simulink model "simulator"  (R2022a)
settings: Solver=FixedStepAuto  StartTime=0.0  StopTime=inf  FixedStep=0.001  RelTol=1e-3
values from neighbouring files (symbols this model uses):
  PWM = [2000;2000;2000;2000]    [startup.m]
undefined symbols (not defined in the file or in its folder): Init, Motor, Vehicle
libraries: matrix_library x2, sldrtlib x1, aerolibnav x1, aerolibanimutils x1, shared6dof x1, sharedtransform x1
settings Model: Creator=Thana  LastModifiedBy=Thana

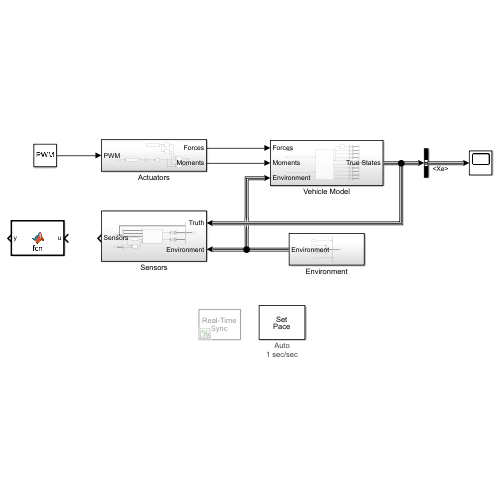
[thumbnail: Simulink's stored preview of the top-level diagram]
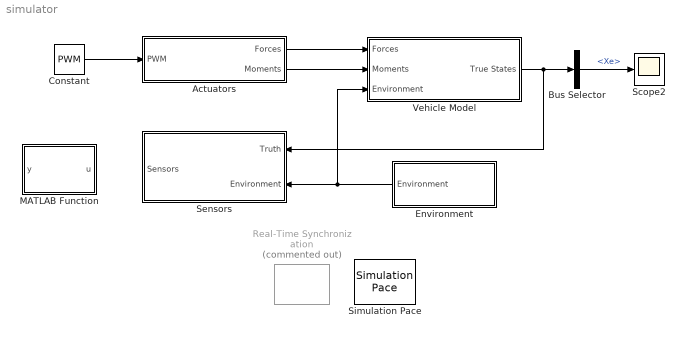
== system simulator ==
  Actuators : Subsystem
  Bus Selector : BusSelector  OutputSignals=Xe
  Constant : Constant  Value=PWM
  Environment : Subsystem
  MATLAB Function : MATLAB Function  TreatAsAtomicUnit=on
  Real-Time Synchronization : sldrtlib/Real-Time Synchronization  Commented=on  SampleTime=1  MaxMissedTicks=1000  ShowMissedTicks=off  YieldWhenWaiting=off
  Scope2 : Scope
  Sensors : Subsystem
  Simulation Pace : aerolibanimutils/Simulation Pace  SimulationPace=1  SleepMode=Auto  OutputPaceError=off  SampleTime=-1
  Vehicle Model : Subsystem
  wires:
  Vehicle Model/1(True States) -> Bus Selector/1, Sensors/1(Truth)
  Environment/1(Environment) -> Vehicle Model/3(Environment), Sensors/2(Environment)
  Actuators/2(Moments) -> Vehicle Model/2(Moments)
  Actuators/1(Forces) -> Vehicle Model/1(Forces)
  Constant/1 -> Actuators/1(PWM)
  Bus Selector/1 -> Scope2/1  "<Xe>"

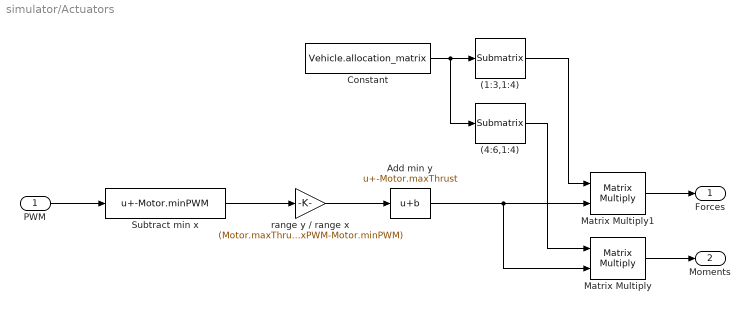
== system simulator/Actuators ==
  PWM : Inport
  (1:3,1:4) : matrix_library/Submatrix  RowSpan=Range of rows  RowStartMode=Index  RowStartIndex=1  RowEndMode=Index  RowEndIndex=3  ColSpan=Range of columns  ColStartMode=Index  ColStartIndex=1  ColEndMode=Index  ColEndIndex=4
      settings: SourceProductBaseCode=SL
  (4:6,1:4) : matrix_library/Submatrix  RowSpan=Range of rows  RowStartMode=Index  RowStartIndex=4  RowEndMode=Index  RowEndIndex=6  ColSpan=Range of columns  ColStartMode=Index  ColStartIndex=1  ColEndMode=Index  ColEndIndex=4
      settings: SourceProductBaseCode=SL
  Add min y : Bias  Bias=-Motor.maxThrust  SaturateOnIntegerOverflow=off
  Constant : Constant  Value=Vehicle.allocation_matrix
  Matrix Multiply : Product  Multiplication=Matrix(*)
  Matrix Multiply1 : Product  Multiplication=Matrix(*)
  Subtract min x : Bias  Bias=-Motor.minPWM  SaturateOnIntegerOverflow=off
  range y / range x : Gain  Gain=(Motor.maxThrust-(-Motor.maxThrust))./(Motor.maxPWM-Motor.minPWM)
  Forces : Outport
  Moments : Outport  Port=2
  wires:
  Add min y/1 -> Matrix Multiply1/2, Matrix Multiply/2
  Subtract min x/1 -> range y / range x/1
  PWM/1 -> Subtract min x/1
  range y / range x/1 -> Add min y/1
  Constant/1 -> (4:6,1:4)/1, (1:3,1:4)/1
  (4:6,1:4)/1 -> Matrix Multiply/1
  (1:3,1:4)/1 -> Matrix Multiply1/1
  Matrix Multiply1/1 -> Forces/1
  Matrix Multiply/1 -> Moments/1

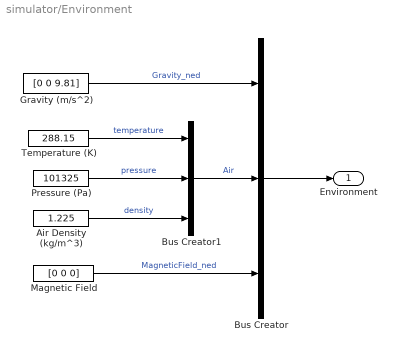
== system simulator/Environment ==
  Air Density (kg/m^3) : Constant  Value=1.225
  Bus Creator : BusCreator  Inputs=3
  Bus Creator1 : BusCreator  Inputs=3
  Gravity (m/s^2) : Constant  Value=[0 0 9.81]
  Magnetic Field : Constant  Value=[0 0 0]
  Pressure (Pa) : Constant  Value=101325
  Temperature (K) : Constant  Value=288.15
  Environment : Outport  VectorParamsAs1DForOutWhenUnconnected=off
  wires:
  Air Density (kg/m^3)/1 -> Bus Creator1/3  "density"
  Bus Creator1/1 -> Bus Creator/2  "Air"
  Bus Creator/1 -> Environment/1
  Pressure (Pa)/1 -> Bus Creator1/2  "pressure"
  Gravity (m/s^2)/1 -> Bus Creator/1  "Gravity_ned"
  Magnetic Field/1 -> Bus Creator/3  "MagneticField_ned"
  Temperature (K)/1 -> Bus Creator1/1  "temperature"

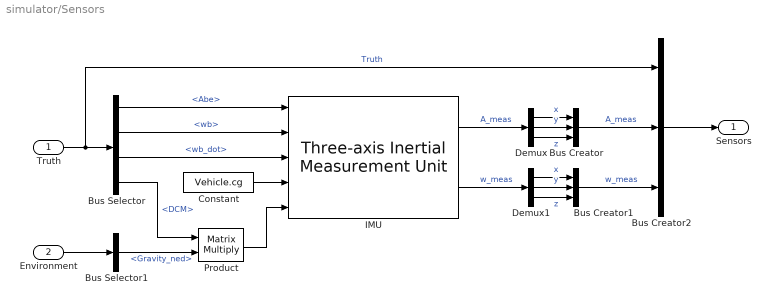
== system simulator/Sensors ==
  Truth : Inport
  Environment : Inport  Port=2
  Bus Creator : BusCreator  Inputs=3
  Bus Creator1 : BusCreator  Inputs=3
  Bus Creator2 : BusCreator  Inputs=3
  Bus Selector : BusSelector  OutputSignals=Abe,wb,wb_dot,DCM
  Bus Selector1 : BusSelector  OutputSignals=Gravity_ned
  Constant : Constant  Value=Vehicle.cg
  Demux : Demux  Outputs=3
  Demux1 : Demux  Outputs=3
  IMU : aerolibnav/Three-axis Inertial Measurement Unit  units=Metric (MKS)  imu=IMU.location  i_Ts=0  dtype_a=on  w_a=190  z_a=0.707  a_sf_cc=[1 0 0; 0 1 0; 0 0 1]  a_bias=[0 0 0]  a_sat="[-inf  -inf  -inf  inf inf inf]"  dtype_g=on  w_g=190  z_g=0.707  g_sf_cc=[1 0 0; 0 1 0; 0 0 1]  g_bias=[0 0 0]  g_sens=[0 0 0]  g_sat="[-inf  -inf  -inf  inf inf inf]"  i_rand=on  i_seeds=[23093 23094 23095 23096 23097 23098]  i_pow=[0.001 0.001 0.001 0.0001 0.0001 0.0001]
  Product : Product  Multiplication=Matrix(*)
  Sensors : Outport
  wires:
  Truth/1 -> Bus Creator2/1, Bus Selector/1  "Truth"
  Bus Selector/1 -> IMU/1  "<Abe>"
  Bus Selector/2 -> IMU/2  "<wb>"
  Bus Selector/3 -> IMU/3  "<wb_dot>"
  Environment/1 -> Bus Selector1/1
  Constant/1 -> IMU/4
  IMU/1 -> Demux/1  "A_meas"
  Demux/1 -> Bus Creator/1  "x"
  Demux/2 -> Bus Creator/2  "y"
  Demux/3 -> Bus Creator/3  "z"
  Demux1/3 -> Bus Creator1/3  "z"
  Demux1/2 -> Bus Creator1/2  "y"
  Demux1/1 -> Bus Creator1/1  "x"
  IMU/2 -> Demux1/1  "w_meas"
  Bus Creator/1 -> Bus Creator2/2  "A_meas"
  Bus Creator1/1 -> Bus Creator2/3  "w_meas"
  Bus Creator2/1 -> Sensors/1
  Bus Selector1/1 -> Product/2  "<Gravity_ned>"
  Bus Selector/4 -> Product/1  "<DCM>"
  Product/1 -> IMU/5

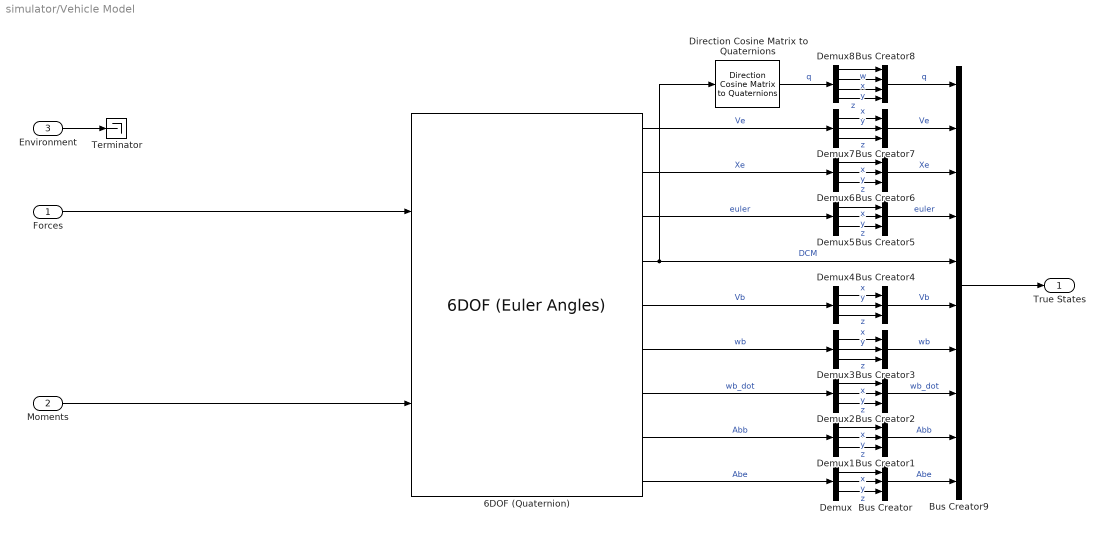
== system simulator/Vehicle Model ==
  Forces : Inport
  Moments : Inport  Port=2
  Environment : Inport  Port=3
  6DOF (Quaternion) : shared6dof/6DOF (Euler Angles)  units=Metric (MKS)  mtype=Fixed  rep=Quaternion  xme_0=[Init.x, Init.y, Init.z]  Vm_0=[Init.u, Init.v, Init.w]  eul_0=[Init.phi, Init.theta, Init.psi]  pm_0=[Init.p, Init.q, Init.r]  mass_0=Vehicle.mass  mass_e=0.5  mass_f=2.0  inertia=Vehicle.inertia  inertia_e=eye(3)  inertia_f=2*eye(3)  k_quat=1.0  vre_flag=on  abi_flag=on  aMode=0  xme_statename=''  Vm_statename=''  eul_statename=''  quat_statename=''  pm_statename=''  mass_statename=''
      settings: SourceProductBaseCode=AE,PW,DR,MT,VE
  Bus Creator{,1..7} (8 alike) : BusCreator  Inputs=3
  Bus Creator8 : BusCreator  Inputs=4
  Bus Creator9 : BusCreator  Inputs=10
  Demux{,1..7} (8 alike) : Demux  Outputs=3
  Demux8 : Demux
  Direction Cosine Matrix to Quaternions : sharedtransform/Direction Cosine Matrix  to Quaternions  aMode=0  action=None  tolerance=eps(2)
      settings: SourceProductBaseCode=AE,PW,DR,MT,VE
  Terminator : Terminator
  True States : Outport
  wires:
  Bus Creator9/1 -> True States/1
  Demux7/1 -> Bus Creator7/1  "x"
  Demux8/4 -> Bus Creator8/4  "z"
  6DOF (Quaternion)/7 -> Demux2/1  "wb_dot"
  Demux6/1 -> Bus Creator6/1  "x"
  Bus Creator8/1 -> Bus Creator9/1  "q"
  Demux4/1 -> Bus Creator4/1  "x"
  Demux6/2 -> Bus Creator6/2  "y"
  Direction Cosine Matrix to Quaternions/1 -> Demux8/1  "q"
  6DOF (Quaternion)/1 -> Demux7/1  "Ve"
  Demux5/3 -> Bus Creator5/3  "z"
  6DOF (Quaternion)/6 -> Demux3/1  "wb"
  Demux8/1 -> Bus Creator8/1  "w"
  Demux/3 -> Bus Creator/3  "z"
  Moments/1 -> 6DOF (Quaternion)/2
  Demux3/2 -> Bus Creator3/2  "y"
  Demux8/3 -> Bus Creator8/3  "y"
  6DOF (Quaternion)/3 -> Demux5/1  "euler"
  Demux2/1 -> Bus Creator2/1  "x"
  Bus Creator2/1 -> Bus Creator9/8  "wb_dot"
  Demux1/3 -> Bus Creator1/3  "z"
  6DOF (Quaternion)/9 -> Demux/1  "Abe"
  Bus Creator/1 -> Bus Creator9/10  "Abe"
  Demux6/3 -> Bus Creator6/3  "z"
  Demux2/2 -> Bus Creator2/2  "y"
  Environment/1 -> Terminator/1
  Bus Creator3/1 -> Bus Creator9/7  "wb"
  Bus Creator4/1 -> Bus Creator9/6  "Vb"
  6DOF (Quaternion)/8 -> Demux1/1  "Abb"
  Bus Creator5/1 -> Bus Creator9/4  "euler"
  Demux2/3 -> Bus Creator2/3  "z"
  Demux5/1 -> Bus Creator5/1  "x"
  Demux4/2 -> Bus Creator4/2  "y"
  Demux7/3 -> Bus Creator7/3  "z"
  Forces/1 -> 6DOF (Quaternion)/1
  Demux7/2 -> Bus Creator7/2  "y"
  Demux1/1 -> Bus Creator1/1  "x"
  Bus Creator6/1 -> Bus Creator9/3  "Xe"
  Demux3/1 -> Bus Creator3/1  "x"
  Demux4/3 -> Bus Creator4/3  "z"
  6DOF (Quaternion)/4 -> Bus Creator9/5, Direction Cosine Matrix to Quaternions/1  "DCM"
  6DOF (Quaternion)/5 -> Demux4/1  "Vb"
  Demux8/2 -> Bus Creator8/2  "x"
  6DOF (Quaternion)/2 -> Demux6/1  "Xe"
  Demux3/3 -> Bus Creator3/3  "z"
  Demux/1 -> Bus Creator/1  "x"
  Bus Creator1/1 -> Bus Creator9/9  "Abb"
  Demux1/2 -> Bus Creator1/2  "y"
  Bus Creator7/1 -> Bus Creator9/2  "Ve"
  Demux5/2 -> Bus Creator5/2  "y"
  Demux/2 -> Bus Creator/2  "y"

== matlab function simulator/MATLAB Function ==
  data: u input; y output
function y = fcn(u)

y = u;
